simulink model "narx_net_Sinusoidal_24_24_6"  (R2019a)
settings: Solver=VariableStepAuto  StartTime=0.0  StopTime=10.0  RelTol=1e-3
libraries: neural x17
(part 2 of 2)

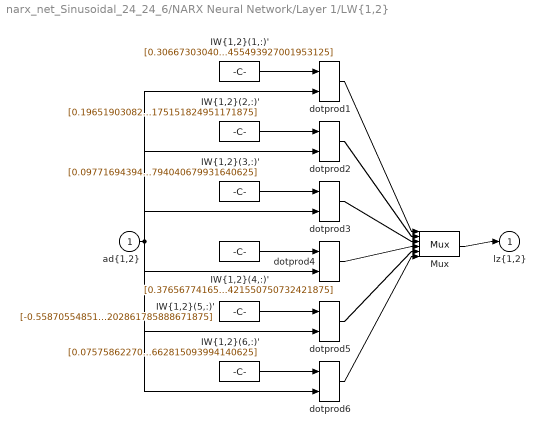
== system narx_net_Sinusoidal_24_24_6/NARX Neural Network/Layer 1/LW{1,2} ==
  "ad{1,2}" : Inport  PortDimensions=24  SampleTime=0.01
      mask Display: e = 0.06;c1 = [120 230 180]/255;c2 = ([120 230 180]+0)/(256+128);c3 = ([120 230 180]+128)/(256+128);patch([0 1 1 0],[0 0 1 1],c1);patch([0 1 1 1-e 1-e 0+e],[0 0 1 1-e 0+e 0+e],c2);patch([0 0 1 1-e 0+e 0+e],[0 1 1 1-e 1-e 0+e],c3);plot([0 1 1 0 0],[0 0 1 1 0]);
  "IW{1,2}(1,:)'" : Constant  Value=[0.306673030408703917171209241132601164281368255615234375;-0.11198177206757127521985495377521147020161151885986328125;0.3269859355907691611520249352906830608844757080078125;0.056270185849424024515652575928470469079911708831787109375;-0.113558622384051233211721410043537616729736328125;0.09782792362847221590005375446708058007061481475830078125;-0.3122359510233196910888864294975064694881439208984375;-0.257081540505827488285461868144921027123928070068359375;0.276391847125739553714396379291429184377193450927734375;0.2222602218884729696757318606614717282354831695556640625;-0.2021395968177663593490223092885571531951427459716796875;0.1814053757736827365842913195592700503766536712646484375;0.2258593327786559690206757977648521773517131805419921875;-0.2029117090672250822702693540122709237039089202880859375;0.0282557608137135353454372221904122852720320224761962890625;-0.230249871903323855004686038228101097047328948974609375;-0.2195438158585874266481852146171149797737598419189453125;0.261170925858878799630247158347629010677337646484375;0.180486427927954939942623013848788104951381683349609375;0.069226347620993278209056143168709240853786468505859375;-0.1443199707426636724250101906363852322101593017578125;-0.2391833789258829556789720527376630343496799468994140625;0.1659067472852251701187498156286892481148242950439453125;0.11194979810412608589587080132332630455493927001953125]
      mask Display: e = 0.06;c1 = [120 150 230]/255;c2 = ([120 150 230]+0)/383;c3 = ([120 150 230]+128)/383;patch([0 1 1 0],[0 0 1 1],c1);patch([0 1 1 1-e 1-e 0+e],[0 0 1 1-e 0+e 0+e],c2);patch([0 0 1 1-e 0+e 0+e],[0 1 1 1-e 1-e 0+e],c3);plot([0 1 1 0 0],[0 0 1 1 0]);disp('weights');
  "IW{1,2}(2,:)'" : Constant  Value=[0.196519030828230689689206656112219206988811492919921875;-0.1595862747555963634393805250510922633111476898193359375;-0.238312071756647425591069122674525715410709381103515625;-0.37667022763899893345040936765144579112529754638671875;-0.01219480248024964845476869612639347906224429607391357421875;-0.16186153809693315519524503542925231158733367919921875;-0.10963349883229563108688608963348087854683399200439453125;0.08577468354507998549163261259309365414083003997802734375;-0.13244028970139598566646554900216870009899139404296875;0.06973027897582433076717478570571984164416790008544921875;0.1996874709654370416700430723722092807292938232421875;0.1414539201875719409695619788180920295417308807373046875;-0.410338678032958481534109296262613497674465179443359375;0.2175943984202941272609876932619954459369182586669921875;0.1394821677224036549080921076892991550266742706298828125;0.0428180467314927259980805729355779476463794708251953125;-0.275353647726182426680452408618293702602386474609375;0.05862862738383915750528529997609439305961132049560546875;0.13762278415745765602906658386928029358386993408203125;-0.136380748418356068096812805379158817231655120849609375;-0.393208750383996219479598721591173671185970306396484375;-0.41983179452645702500745983343222178518772125244140625;0.0193259477496929565898398095669108442962169647216796875;0.051822453742941747278916153618411044590175151824951171875]
      mask Display: e = 0.06;c1 = [120 150 230]/255;c2 = ([120 150 230]+0)/383;c3 = ([120 150 230]+128)/383;patch([0 1 1 0],[0 0 1 1],c1);patch([0 1 1 1-e 1-e 0+e],[0 0 1 1-e 0+e 0+e],c2);patch([0 0 1 1-e 0+e 0+e],[0 1 1 1-e 1-e 0+e],c3);plot([0 1 1 0 0],[0 0 1 1 0]);disp('weights');
  "IW{1,2}(3,:)'" : Constant  Value=[0.09771694394740902678275773496352485381066799163818359375;-0.1415025473628825636307482227493892423808574676513671875;0.1755285439126030022638502714471542276442050933837890625;0.1116232255050156052522680738547933287918567657470703125;-0.34408022982841279802102008034125901758670806884765625;0.0792148754280949385364607451265328563749790191650390625;0.266739206129793571253827622058452107012271881103515625;0.2537797995477009127540668487199582159519195556640625;0.305212184974735178943916480420739389955997467041015625;-0.3149703916652015767141392643679864704608917236328125;0.264525796061264750758112995754345320165157318115234375;-0.2530632579431484341370151014416478574275970458984375;0.025395663220353130451467649209007504396140575408935546875;0.2409238223387252519902546055163838900625705718994140625;0.32858810067802923793323088830220513045787811279296875;-0.261318748295446268148367607864202000200748443603515625;0.1881791957386545754982165590263321064412593841552734375;-0.10850413491654682662801434389621135778725147247314453125;0.2217647526361911924919212424356373958289623260498046875;-0.31005730369838302440399502302170731127262115478515625;0.05467111885891319522645659390036598779261112213134765625;0.210146756312323101933969837773474864661693572998046875;0.341591394286220928488972958803060464560985565185546875;0.17273883000019341071862299941130913794040679931640625]
      mask Display: e = 0.06;c1 = [120 150 230]/255;c2 = ([120 150 230]+0)/383;c3 = ([120 150 230]+128)/383;patch([0 1 1 0],[0 0 1 1],c1);patch([0 1 1 1-e 1-e 0+e],[0 0 1 1-e 0+e 0+e],c2);patch([0 0 1 1-e 0+e 0+e],[0 1 1 1-e 1-e 0+e],c3);plot([0 1 1 0 0],[0 0 1 1 0]);disp('weights');
  "IW{1,2}(4,:)'" : Constant  Value=[0.376567741656371468561559368026792071759700775146484375;-0.226796412015716819521315983365639112889766693115234375;0.1288925676318834756539644104122999124228954315185546875;-0.0703574015836986033090028058722964487969875335693359375;0.036116553042721107058543594803268206305801868438720703125;0.00456047255372171549125948075698033790104091167449951171875;-0.003630385408504195610124298809751053340733051300048828125;0.016596451191842331862602577530196867883205413818359375;0.007788283319363454963724091584253983455710113048553466796875;-0.01299859135048583337612715382647365913726389408111572265625;0.01145889041297005160602306972350561409257352352142333984375;-0.01316943770400048896451750124469981528818607330322265625;0.018599606798864846968211139710547286085784435272216796875;0.0029078928036930192825570973269577734754420816898345947265625;-0.00020205609617424431377792626296496791837853379547595977783203125;-0.007535644507239321054914427122639608569443225860595703125;0.00942303876382953424506450090802900376729667186737060546875;-0.0306685189480544635742820247514828224666416645050048828125;0.0431527151917643070344610123356687836349010467529296875;-0.03292662848017215149187819633880280889570713043212890625;0.0289622948350503235659392231582387466914951801300048828125;-0.0157427143958187194805464770297476206906139850616455078125;0.01559357247640663461651922006012682686559855937957763671875;-0.0123741206487570643002271708610351197421550750732421875]
      mask Display: e = 0.06;c1 = [120 150 230]/255;c2 = ([120 150 230]+0)/383;c3 = ([120 150 230]+128)/383;patch([0 1 1 0],[0 0 1 1],c1);patch([0 1 1 1-e 1-e 0+e],[0 0 1 1-e 0+e 0+e],c2);patch([0 0 1 1-e 0+e 0+e],[0 1 1 1-e 1-e 0+e],c3);plot([0 1 1 0 0],[0 0 1 1 0]);disp('weights');
  "IW{1,2}(5,:)'" : Constant  Value=[-0.55870554851228948489705317115294747054576873779296875;0.07272659225011755823597781045464216731488704681396484375;0.054468456770181673809450018097777501679956912994384765625;-0.08931506060536253954751373385079205036163330078125;0.03757319402559498866533971295211813412606716156005859375;0.033882810130841621576447408870080835185945034027099609375;-0.0316717851875283062934585132097708992660045623779296875;0.034115471430612130665505077331545180641114711761474609375;0.039509450488714951965629751384767587296664714813232421875;-0.08457828136277301123158167683868668973445892333984375;0.0684207651316723064471858606339083053171634674072265625;-0.05757860294501955522594727199248154647648334503173828125;0.05457062570232155962468567622636328451335430145263671875;0.00171703879725057842985103118138567879213951528072357177734375;-0.0104754842807108887459133228503560530953109264373779296875;-0.022728858084237961445506215341083589009940624237060546875;0.046300541575451915898842258911827229894697666168212890625;-0.11998735138502857056064243579385220073163509368896484375;0.16380339683133848804885701611055992543697357177734375;-0.1380869937040725137222807461512275040149688720703125;0.113004389650570191694356481093564070761203765869140625;-0.0573476784986787502251814885312342084944248199462890625;0.035521598388957374703434055618345155380666255950927734375;-0.049287448855453823426397974571955273859202861785888671875]
      mask Display: e = 0.06;c1 = [120 150 230]/255;c2 = ([120 150 230]+0)/383;c3 = ([120 150 230]+128)/383;patch([0 1 1 0],[0 0 1 1],c1);patch([0 1 1 1-e 1-e 0+e],[0 0 1 1-e 0+e 0+e],c2);patch([0 0 1 1-e 0+e 0+e],[0 1 1 1-e 1-e 0+e],c3);plot([0 1 1 0 0],[0 0 1 1 0]);disp('weights');
  "IW{1,2}(6,:)'" : Constant  Value=[0.0757586227050215388345577594009228050708770751953125;-0.27684473270092035956935205831541679799556732177734375;0.264526169646414455183247582681360654532909393310546875;-0.2888354913074187013677374125109054148197174072265625;-0.3042240724428435516557556184125132858753204345703125;0.2296829497905580608207998238867730833590030670166015625;0.09251050887686319834646297977087670005857944488525390625;0.37829873239017264285877217844245024025440216064453125;0.06326772721295646773054244249578914605081081390380859375;0.19124998334157528034893402946181595325469970703125;0.04753677910932539718569245223989128135144710540771484375;0.015009511298633780584932395640862523578107357025146484375;0.07473145941779786582959133056647260673344135284423828125;0.2185796547470139350455298199449316598474979400634765625;0.335696523217766384927784883984713815152645111083984375;-0.1889761753167945868003840814708382822573184967041015625;-0.2552293769360109987331952652311883866786956787109375;0.169419213418987746333499444517656229436397552490234375;-0.03779132130635280695241107196125085465610027313232421875;0.0046226941957490420842535883139134966768324375152587890625;-0.031016369668211217491826658942954964004456996917724609375;-0.319486968289223849382096886984072625637054443359375;0.2340934549271946607529315542706171981990337371826171875;-0.33456530111625470969016760136582888662815093994140625]
      mask Display: e = 0.06;c1 = [120 150 230]/255;c2 = ([120 150 230]+0)/383;c3 = ([120 150 230]+128)/383;patch([0 1 1 0],[0 0 1 1],c1);patch([0 1 1 1-e 1-e 0+e],[0 0 1 1-e 0+e 0+e],c2);patch([0 0 1 1-e 0+e 0+e],[0 1 1 1-e 1-e 0+e],c3);plot([0 1 1 0 0],[0 0 1 1 0]);disp('weights');
  Mux : Mux  Inputs=6
      mask Display: e = 0.06;c1 = [120 150 230]/255;c2 = ([120 150 230]+0)/383;c3 = ([120 150 230]+128)/383;patch([0 1 1 0],[0 0 1 1],c1);patch([0 1 1 1-e 1-e 0+e],[0 0 1 1-e 0+e 0+e],c2);patch([0 0 1 1-e 0+e 0+e],[0 1 1 1-e 1-e 0+e],c3);plot([0 1 1 0 0],[0 0 1 1 0]);disp('Mux');
  dotprod{1..6} (6 alike) : neural/Weight Functions/dotprod
      settings: SourceProductName=MATLAB Runtime - Deep Learning Toolbox  SourceProductBaseCode=Missing
  "lz{1,2}" : Outport
      mask Display: e = 0.06;c1 = [120 230 180]/255;c2 = ([120 230 180]+0)/(256+128);c3 = ([120 230 180]+128)/(256+128);patch([0 1 1 0],[0 0 1 1],c1);patch([0 1 1 1-e 1-e 0+e],[0 0 1 1-e 0+e 0+e],c2);patch([0 0 1 1-e 0+e 0+e],[0 1 1 1-e 1-e 0+e],c3);plot([0 1 1 0 0],[0 0 1 1 0]);
  wires:
  "IW{1,2}(1,:)'"/1 -> dotprod1/1
  "ad{1,2}"/1 -> dotprod1/2, dotprod2/2, dotprod3/2, dotprod4/2, dotprod5/2, dotprod6/2
  dotprod1/1 -> Mux/1
  "IW{1,2}(2,:)'"/1 -> dotprod2/1
  dotprod2/1 -> Mux/2
  "IW{1,2}(3,:)'"/1 -> dotprod3/1
  dotprod3/1 -> Mux/3
  "IW{1,2}(4,:)'"/1 -> dotprod4/1
  dotprod4/1 -> Mux/4
  "IW{1,2}(5,:)'"/1 -> dotprod5/1
  dotprod5/1 -> Mux/5
  "IW{1,2}(6,:)'"/1 -> dotprod6/1
  dotprod6/1 -> Mux/6
  Mux/1 -> "lz{1,2}"/1

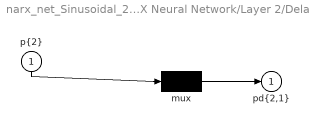
== system narx_net_Sinusoidal_24_24_6/NARX Neural Network/Layer 2/Delays 1 ==
  "p{2}" : Inport  PortDimensions=6  SampleTime=0.01
      mask Display: e = 0.06;c1 = [120 230 180]/255;c2 = ([120 230 180]+0)/(256+128);c3 = ([120 230 180]+128)/(256+128);patch([0 1 1 0],[0 0 1 1],c1);patch([0 1 1 1-e 1-e 0+e],[0 0 1 1-e 0+e 0+e],c2);patch([0 0 1 1-e 0+e 0+e],[0 1 1 1-e 1-e 0+e],c3);plot([0 1 1 0 0],[0 0 1 1 0]);
  mux : Mux  Inputs=1
      mask Display: e = 0.06;c1 = [120 150 230]/255;c2 = ([120 150 230]+0)/383;c3 = ([120 150 230]+128)/383;patch([0 1 1 0],[0 0 1 1],c1);patch([0 1 1 1-e 1-e 0+e],[0 0 1 1-e 0+e 0+e],c2);patch([0 0 1 1-e 0+e 0+e],[0 1 1 1-e 1-e 0+e],c3);plot([0 1 1 0 0],[0 0 1 1 0]);disp('Mux')
  "pd{2,1}" : Outport
      mask Display: e = 0.06;c1 = [120 230 180]/255;c2 = ([120 230 180]+0)/(256+128);c3 = ([120 230 180]+128)/(256+128);patch([0 1 1 0],[0 0 1 1],c1);patch([0 1 1 1-e 1-e 0+e],[0 0 1 1-e 0+e 0+e],c2);patch([0 0 1 1-e 0+e 0+e],[0 1 1 1-e 1-e 0+e],c3);plot([0 1 1 0 0],[0 0 1 1 0]);
  wires:
  "p{2}"/1 -> mux/1
  mux/1 -> "pd{2,1}"/1

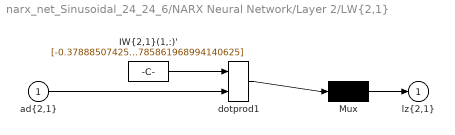
== system narx_net_Sinusoidal_24_24_6/NARX Neural Network/Layer 2/LW{2,1} ==
  "ad{2,1}" : Inport  PortDimensions=6  SampleTime=0.01
      mask Display: e = 0.06;c1 = [120 230 180]/255;c2 = ([120 230 180]+0)/(256+128);c3 = ([120 230 180]+128)/(256+128);patch([0 1 1 0],[0 0 1 1],c1);patch([0 1 1 1-e 1-e 0+e],[0 0 1 1-e 0+e 0+e],c2);patch([0 0 1 1-e 0+e 0+e],[0 1 1 1-e 1-e 0+e],c3);plot([0 1 1 0 0],[0 0 1 1 0]);
  "IW{2,1}(1,:)'" : Constant  Value=[-0.378885074258745568887007948433165438473224639892578125;0.002013940415117906716779838660613677348010241985321044921875;0.001397711243469999635447020835954390349797904491424560546875;3.04057341128410474340171276708133518695831298828125;-1.10259388683669801167752666515298187732696533203125;0.000710811807877522795241775899199865307309664785861968994140625]
      mask Display: e = 0.06;c1 = [120 150 230]/255;c2 = ([120 150 230]+0)/383;c3 = ([120 150 230]+128)/383;patch([0 1 1 0],[0 0 1 1],c1);patch([0 1 1 1-e 1-e 0+e],[0 0 1 1-e 0+e 0+e],c2);patch([0 0 1 1-e 0+e 0+e],[0 1 1 1-e 1-e 0+e],c3);plot([0 1 1 0 0],[0 0 1 1 0]);disp('weights');
  Mux : Mux  Inputs=1
      mask Display: e = 0.06;c1 = [120 150 230]/255;c2 = ([120 150 230]+0)/383;c3 = ([120 150 230]+128)/383;patch([0 1 1 0],[0 0 1 1],c1);patch([0 1 1 1-e 1-e 0+e],[0 0 1 1-e 0+e 0+e],c2);patch([0 0 1 1-e 0+e 0+e],[0 1 1 1-e 1-e 0+e],c3);plot([0 1 1 0 0],[0 0 1 1 0]);disp('Mux');
  dotprod1 : neural/Weight Functions/dotprod
      settings: SourceProductName=MATLAB Runtime - Deep Learning Toolbox  SourceProductBaseCode=Missing
  "lz{2,1}" : Outport
      mask Display: e = 0.06;c1 = [120 230 180]/255;c2 = ([120 230 180]+0)/(256+128);c3 = ([120 230 180]+128)/(256+128);patch([0 1 1 0],[0 0 1 1],c1);patch([0 1 1 1-e 1-e 0+e],[0 0 1 1-e 0+e 0+e],c2);patch([0 0 1 1-e 0+e 0+e],[0 1 1 1-e 1-e 0+e],c3);plot([0 1 1 0 0],[0 0 1 1 0]);
  wires:
  "IW{2,1}(1,:)'"/1 -> dotprod1/1
  "ad{2,1}"/1 -> dotprod1/2
  dotprod1/1 -> Mux/1
  Mux/1 -> "lz{2,1}"/1
